simulink model "PitchHeave"  (R2014a)
settings: Solver=ode45  StartTime=0.0  StopTime=20  RelTol=1e-3
settings Model: Creator=thortom12  LastModifiedBy=thortom12
settings DebuggingCC: SolverPrmCheckMsg=none

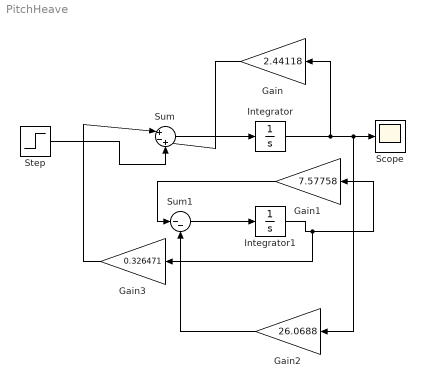
== system PitchHeave ==
  Gain : Gain  Gain=2.44118
  Gain1 : Gain  Gain=7.57758
  Gain2 : Gain  Gain=26.0688
  Gain3 : Gain  Gain=0.326471
  Integrator : Integrator
  Integrator1 : Integrator
  Scope : Scope
  Step : Step  SampleTime=0
  Sum : Sum  Inputs=|+-+
  Sum1 : Sum  Inputs=|--
  wires:
  Gain/1 -> Sum/2
  Sum/1 -> Integrator/1
  Integrator/1 -> Gain/1, Gain2/1, Scope/1
  Sum1/1 -> Integrator1/1
  Integrator1/1 -> Gain3/1, Gain1/1
  Gain1/1 -> Sum1/1
  Gain2/1 -> Sum1/2
  Gain3/1 -> Sum/1
  Step/1 -> Sum/3
